simulink model "Client"  (R2021a)
settings: Solver=ode2  StartTime=0.0  StopTime=inf  FixedStep=0.002  RelTol=1e-3  EnableMultiTasking=on
libraries: quarc_library x19, simulink_extras x6, pid_lib x6, simulink x3
settings Model: SimulationMode=external  ExtModeTrigDuration=10000  Creator=user  LastModifiedBy=user
settings SolverCC: AlgebraicLoopSolver=TrustRegion  PositivePriorityOrder=on
settings DataIOCC: ReturnWorkspaceOutputs=off
settings DebuggingCC: SFMachineParentedDataDiag=warning  ArithmeticOperatorsInVariantConditions=warning
settings SFSimCC: SimUseLocalCustomCode=off  CustomCodeUndefinedFunction=UseInterfaceOnly
settings RTWCC: Description=QUARC Win64 Target Using Toolchain  SystemTargetFile=quarc_win64.tlc  TemplateMakefile=quarc_default_tmf  RTWUseLocalCustomCode=off  Toolchain=QUARC win64 | nmake (64-bit Windows)  BuildConfiguration=Faster Runs
settings CodeAppCC: StateflowObjectComments=on
settings STFCustomTargetCC: TargetLangStandard=C99 (ISO)  ConcurrentExecutionCompliant=on  SystemTargetFile=quarc_win64.tlc
settings GRTTargetCC: ParMdlRefBuildCompliant=off  CompOptLevelCompliant=off  CombineOutputUpdateFcns=off  MatFileLogging=off  CPPClassGenCompliant=off  GRTInterface=on  ExtMode=on  ExtModeMexFile=quarc_comm  ExtModeMexArgs='-w -d /tmp -uri %u','tcpip://localhost:17001'
settings ConfigComp: CovMetricSettings=dswe

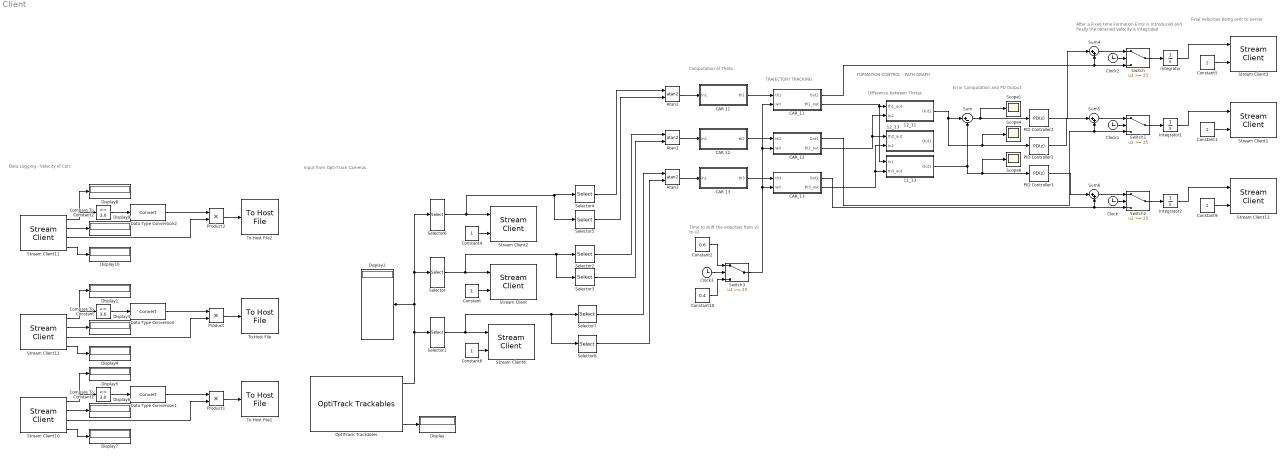
== system Client ==
  note: TRAJECTORY TRACKING
  note: FORMATION CONTROL - PATH GRAPH
  note: Difference between Thetas
  note: Error Computation and PD Output
  note: After a Fixed time Formation Error is
      | Introduced and finally the obtained
      | velocity is integrated
  note: Final Velocities being sent
      | to Server
  note: TIme to shift the velocities
      | from v1 to v2
  note: Computation of Theta
  note: Input from Opti-Track Cameras
  note: Data Logging - Velocity of Cars
  11_13 : Subsystem
  12_11 : Subsystem
  12_13 : Subsystem
  Atan1 : Trigonometry  Operator=atan2
  Atan2 : Trigonometry  Operator=atan2
  Atan3 : Trigonometry  Operator=atan2
  CAR 11 : Subsystem
  CAR 12 : Subsystem
  CAR 13 : Subsystem
  CAR_11 : Subsystem
  CAR_12 : Subsystem
  CAR_13 : Subsystem
  Clock{,1..3} (4 alike) : Clock
  Compare To Constant : simulink/Logic and Bit Operations/Compare To Constant  relop=<=  const=3.0  OutDataTypeStr=boolean
  Compare To Constant1 : simulink/Logic and Bit Operations/Compare To Constant  relop=<=  const=3.0  OutDataTypeStr=boolean
  Compare To Constant2 : simulink/Logic and Bit Operations/Compare To Constant  relop=<=  const=3.0  OutDataTypeStr=boolean
  Constant{,1,4..6,9} (6 alike) : Constant
  Constant10 : Constant  Value=0.4
  Constant2 : Constant  Value=0.6
  Data Type Conversion : DataTypeConversion
  Data Type Conversion1 : DataTypeConversion
  Data Type Conversion2 : DataTypeConversion
  Display{,1..10} (11 alike) : Display
  Integrator : Integrator  LimitOutput=on  UpperSaturationLimit=5  LowerSaturationLimit=0  WrappedStateUpperValue=5  WrappedStateLowerValue=0
  Integrator1 : Integrator  LimitOutput=on  UpperSaturationLimit=5  LowerSaturationLimit=0
  Integrator2 : Integrator  LimitOutput=on  UpperSaturationLimit=5  LowerSaturationLimit=0
  OptiTrack Trackables : quarc_library/Devices/Third-Party/NaturalPoint/OptiTrack/OptiTrack Trackables  calibration_file=C:\Users\user\Desktop\Motive_Calibration_SingleDrone\Camera_Calibration_Training\Calibration Exceptional (MeanErr 0.434 mm) 2023-02-26 3.cal  rigid_body_file=C:\Users\user\Desktop\Motive_Calibration_SingleDrone\Camera_Calibration_Training\3 Cars_1.tra  rigid_body_ids=[5 6 7]  sample_time=qc_get_step_size  active=off
      settings: SourceProductName=QUARC Targets
  PID Controller1 : pid_lib/PID Controller  Controller=PD  Form=Parallel  TimeDomain=Discrete-time  UseExternalTs=off  SampleTime=-1  IntegratorMethod=Forward Euler  FilterMethod=Forward Euler  ControllerParametersSource=internal  P=-0.68  I=-0.5  D=-1.75  UseFilter=on  N=1  TunerSelectOption=Transfer Function Based (PID Tuner App)  InitialConditionSource=internal  InitialConditionForIntegrator=0  InitialConditionForFilter=0  DifferentiatorICPrevScaledInput=0  ExternalReset=none  TrackingMode=off  Kt=1  LimitOutput=off  SatLimitsSource=internal  UpperSaturationLimit=inf  LowerSaturationLimit=-inf  LinearizeAsGain=on  AntiWindupMode=none  Kb=1  POutMin=[]  POutMax=[]  IOutMin=[]  IOutMax=[]  DOutMin=[]  DOutMax=[]  NOutMin=[]  NOutMax=[]  SumOutMin=[]  SumOutMax=[]  SaturationOutMin=[]  SaturationOutMax=[]  PParamMin=[]  PParamMax=[]  IParamMin=[]  IParamMax=[]  DParamMin=[]  DParamMax=[]  NParamMin=[]  NParamMax=[]  KbParamMin=[]  KbParamMax=[]  KtParamMin=[]  KtParamMax=[]  KbOutMin=[]  KbOutMax=[]  KtOutMin=[]  KtOutMax=[]  IntegratorOutMin=[]  IntegratorOutMax=[]  FilterOutMin=[]  FilterOutMax=[]  SumI1OutMin=[]  SumI1OutMax=[]  SumI2OutMin=[]  SumI2OutMax=[]  SumI3OutMin=[]  SumI3OutMax=[]  SumI4OutMin=[]  SumI4OutMax=[]  SumDOutMin=[]  SumDOutMax=[]  DifferentiatorOutMin=[]  DifferentiatorOutMax=[]  FilterDiffOutCoefMin=[]  FilterDiffOutCoefMax=[]  ReciprocalOutMin=[]  ReciprocalOutMax=[]  SumDenOutMin=[]  SumDenOutMax=[]  SumNumOutMin=[]  SumNumOutMax=[]  DivideOutMin=[]  DivideOutMax=[]  UdiffTsProdOutMin=[]  UdiffTsProdOutMax=[]  NTsProdOutMin=[]  NTsProdOutMax=[]  UintegralTsProdOutMin=[]  UintegralTsProdOutMax=[]  UngainTsProdOutMin=[]  UngainTsProdOutMax=[]  IntegratorContinuousStateAttributes=''  IntegratorStateMustResolveToSignalObject=off  IntegratorRTWStateStorageClass=Auto  FilterContinuousStateAttributes=''  FilterStateMustResolveToSignalObject=off  FilterRTWStateStorageClass=Auto  ParallelPVariant=InternalParameters  IdealPVariant=Disabled  IVariant=Disabled  DVariant=InternalParameters  IntegratorVariant=Disabled  SatVariant=Disabled  AWVariant=Disabled  PCopyVariant=Disabled  TRVariant=Disabled  FdbkBlocksVariant=Forward  IdealPFdbkVariant=Disabled  SatFdbkVariant=Disabled  DerivativeFilterVariant=ForwardEulerFilter  NVariant=InternalParameters  NCopyVariant=Disabled  FilterICVariant=InternalICsFilter  IntegratorICVariant=Disabled  ExternalResetVariant=Disabled  TRSumVariant=Passthrough  SumFdbkVariant=Disabled  SumVariant=Sum_PD  TsampFilterVariant=InternalTs  TsampNgainVariant=Passthrough  TsampIntegralVariant=Disabled_SignalSpec  ExternalSaturationOutDataTypeStr=Inherit: Same as second input
  PID Controller2 : pid_lib/PID Controller  Controller=PD  Form=Parallel  TimeDomain=Discrete-time  UseExternalTs=off  SampleTime=-1  IntegratorMethod=Forward Euler  FilterMethod=Forward Euler  ControllerParametersSource=internal  P=-0.68  I=-0.5  D=-1.75  UseFilter=on  N=1  TunerSelectOption=Transfer Function Based (PID Tuner App)  InitialConditionSource=internal  InitialConditionForIntegrator=0  InitialConditionForFilter=0  DifferentiatorICPrevScaledInput=0  ExternalReset=none  TrackingMode=off  Kt=1  LimitOutput=off  SatLimitsSource=internal  UpperSaturationLimit=inf  LowerSaturationLimit=-inf  LinearizeAsGain=on  AntiWindupMode=none  Kb=1  POutMin=[]  POutMax=[]  IOutMin=[]  IOutMax=[]  DOutMin=[]  DOutMax=[]  NOutMin=[]  NOutMax=[]  SumOutMin=[]  SumOutMax=[]  SaturationOutMin=[]  SaturationOutMax=[]  PParamMin=[]  PParamMax=[]  IParamMin=[]  IParamMax=[]  DParamMin=[]  DParamMax=[]  NParamMin=[]  NParamMax=[]  KbParamMin=[]  KbParamMax=[]  KtParamMin=[]  KtParamMax=[]  KbOutMin=[]  KbOutMax=[]  KtOutMin=[]  KtOutMax=[]  IntegratorOutMin=[]  IntegratorOutMax=[]  FilterOutMin=[]  FilterOutMax=[]  SumI1OutMin=[]  SumI1OutMax=[]  SumI2OutMin=[]  SumI2OutMax=[]  SumI3OutMin=[]  SumI3OutMax=[]  SumI4OutMin=[]  SumI4OutMax=[]  SumDOutMin=[]  SumDOutMax=[]  DifferentiatorOutMin=[]  DifferentiatorOutMax=[]  FilterDiffOutCoefMin=[]  FilterDiffOutCoefMax=[]  ReciprocalOutMin=[]  ReciprocalOutMax=[]  SumDenOutMin=[]  SumDenOutMax=[]  SumNumOutMin=[]  SumNumOutMax=[]  DivideOutMin=[]  DivideOutMax=[]  UdiffTsProdOutMin=[]  UdiffTsProdOutMax=[]  NTsProdOutMin=[]  NTsProdOutMax=[]  UintegralTsProdOutMin=[]  UintegralTsProdOutMax=[]  UngainTsProdOutMin=[]  UngainTsProdOutMax=[]  IntegratorContinuousStateAttributes=''  IntegratorStateMustResolveToSignalObject=off  IntegratorRTWStateStorageClass=Auto  FilterContinuousStateAttributes=''  FilterStateMustResolveToSignalObject=off  FilterRTWStateStorageClass=Auto  ParallelPVariant=InternalParameters  IdealPVariant=Disabled  IVariant=Disabled  DVariant=InternalParameters  IntegratorVariant=Disabled  SatVariant=Disabled  AWVariant=Disabled  PCopyVariant=Disabled  TRVariant=Disabled  FdbkBlocksVariant=Forward  IdealPFdbkVariant=Disabled  SatFdbkVariant=Disabled  DerivativeFilterVariant=ForwardEulerFilter  NVariant=InternalParameters  NCopyVariant=Disabled  FilterICVariant=InternalICsFilter  IntegratorICVariant=Disabled  ExternalResetVariant=Disabled  TRSumVariant=Passthrough  SumFdbkVariant=Disabled  SumVariant=Sum_PD  TsampFilterVariant=InternalTs  TsampNgainVariant=Passthrough  TsampIntegralVariant=Disabled_SignalSpec  ExternalSaturationOutDataTypeStr=Inherit: Same as second input
  PID Controller3 : pid_lib/PID Controller  Controller=PD  Form=Parallel  TimeDomain=Discrete-time  UseExternalTs=off  SampleTime=-1  IntegratorMethod=Forward Euler  FilterMethod=Forward Euler  ControllerParametersSource=internal  P=-0.68  I=-0.5  D=-1.75  UseFilter=on  N=1  TunerSelectOption=Transfer Function Based (PID Tuner App)  InitialConditionSource=internal  InitialConditionForIntegrator=0  InitialConditionForFilter=0  DifferentiatorICPrevScaledInput=0  ExternalReset=none  TrackingMode=off  Kt=1  LimitOutput=off  SatLimitsSource=internal  UpperSaturationLimit=inf  LowerSaturationLimit=-inf  LinearizeAsGain=on  AntiWindupMode=none  Kb=1  POutMin=[]  POutMax=[]  IOutMin=[]  IOutMax=[]  DOutMin=[]  DOutMax=[]  NOutMin=[]  NOutMax=[]  SumOutMin=[]  SumOutMax=[]  SaturationOutMin=[]  SaturationOutMax=[]  PParamMin=[]  PParamMax=[]  IParamMin=[]  IParamMax=[]  DParamMin=[]  DParamMax=[]  NParamMin=[]  NParamMax=[]  KbParamMin=[]  KbParamMax=[]  KtParamMin=[]  KtParamMax=[]  KbOutMin=[]  KbOutMax=[]  KtOutMin=[]  KtOutMax=[]  IntegratorOutMin=[]  IntegratorOutMax=[]  FilterOutMin=[]  FilterOutMax=[]  SumI1OutMin=[]  SumI1OutMax=[]  SumI2OutMin=[]  SumI2OutMax=[]  SumI3OutMin=[]  SumI3OutMax=[]  SumI4OutMin=[]  SumI4OutMax=[]  SumDOutMin=[]  SumDOutMax=[]  DifferentiatorOutMin=[]  DifferentiatorOutMax=[]  FilterDiffOutCoefMin=[]  FilterDiffOutCoefMax=[]  ReciprocalOutMin=[]  ReciprocalOutMax=[]  SumDenOutMin=[]  SumDenOutMax=[]  SumNumOutMin=[]  SumNumOutMax=[]  DivideOutMin=[]  DivideOutMax=[]  UdiffTsProdOutMin=[]  UdiffTsProdOutMax=[]  NTsProdOutMin=[]  NTsProdOutMax=[]  UintegralTsProdOutMin=[]  UintegralTsProdOutMax=[]  UngainTsProdOutMin=[]  UngainTsProdOutMax=[]  IntegratorContinuousStateAttributes=''  IntegratorStateMustResolveToSignalObject=off  IntegratorRTWStateStorageClass=Auto  FilterContinuousStateAttributes=''  FilterStateMustResolveToSignalObject=off  FilterRTWStateStorageClass=Auto  ParallelPVariant=InternalParameters  IdealPVariant=Disabled  IVariant=Disabled  DVariant=InternalParameters  IntegratorVariant=Disabled  SatVariant=Disabled  AWVariant=Disabled  PCopyVariant=Disabled  TRVariant=Disabled  FdbkBlocksVariant=Forward  IdealPFdbkVariant=Disabled  SatFdbkVariant=Disabled  DerivativeFilterVariant=ForwardEulerFilter  NVariant=InternalParameters  NCopyVariant=Disabled  FilterICVariant=InternalICsFilter  IntegratorICVariant=Disabled  ExternalResetVariant=Disabled  TRSumVariant=Passthrough  SumFdbkVariant=Disabled  SumVariant=Sum_PD  TsampFilterVariant=InternalTs  TsampNgainVariant=Passthrough  TsampIntegralVariant=Disabled_SignalSpec  ExternalSaturationOutDataTypeStr=Inherit: Same as second input
  Product : Product
  Product1 : Product
  Product2 : Product
  Scope1 : Scope
  Scope4 : Scope
  Scope6 : Scope
  Selector : Selector  InputPortWidth=9  IndexOptions=Index vector (dialog)  Indices=[1 3]  OutputSizes=1
  Selector1 : Selector  InputPortWidth=9  IndexOptions=Index vector (dialog)  Indices=[7 9]  OutputSizes=1
  Selector2 : Selector  InputPortWidth=2  IndexOptions=Index vector (dialog)  Indices=[1]  OutputSizes=1
  Selector3 : Selector  InputPortWidth=2  IndexOptions=Index vector (dialog)  Indices=[2]  OutputSizes=1
  Selector4 : Selector  InputPortWidth=2  IndexOptions=Index vector (dialog)  Indices=[1]  OutputSizes=1
  Selector5 : Selector  InputPortWidth=2  IndexOptions=Index vector (dialog)  Indices=[2]  OutputSizes=1
  Selector6 : Selector  InputPortWidth=9  IndexOptions=Index vector (dialog)  Indices=[4 6]  OutputSizes=1
  Selector7 : Selector  InputPortWidth=2  IndexOptions=Index vector (dialog)  Indices=[1]  OutputSizes=1
  Selector8 : Selector  InputPortWidth=2  IndexOptions=Index vector (dialog)  Indices=[2]  OutputSizes=1
  Stream Client : quarc_library/Communications/Basic/Stream Client  uri_source=Specify via dialog (do not evaluate)  uri=tcpip://192.168.2.12:18070  send_buffer_size=1460  receive_buffer_size=1460  byte_order=little endian (Intel - LSB first)  optimization=Minimum latency  send_options=Send most recent data  receive_options=Do not receive data  default_value=[0]  sample_time=qc_get_step_size  active=off  implementation=Use blocking I/O in a separate thread  send_fifo_size=1000  receive_fifo_size=1000  send_priority=0  receive_priority=0  send_dimensions=off  receive_dimensions=off  max_dimensions=-1  data_type=Inherited via back propagation  type_expr=BusObject
      settings: AttributesFormatString="\"tcpip://192.168.2.12:18070\""
  Stream Client1 : quarc_library/Communications/Basic/Stream Client  uri_source=Specify via dialog (do not evaluate)  uri=tcpip://192.168.2.12:18071  send_buffer_size=1460  receive_buffer_size=1460  byte_order=little endian (Intel - LSB first)  optimization=Minimum latency  send_options=Send most recent data  receive_options=Do not receive data  default_value=[0]  sample_time=qc_get_step_size  active=off  implementation=Use blocking I/O in a separate thread  send_fifo_size=1000  receive_fifo_size=1000  send_priority=0  receive_priority=0  send_dimensions=off  receive_dimensions=off  max_dimensions=-1  data_type=Inherited via back propagation  type_expr=BusObject
      settings: AttributesFormatString="\"tcpip://192.168.2.12:18071\""
  Stream Client10 : quarc_library/Communications/Basic/Stream Client  uri_source=Specify via dialog (do not evaluate)  uri=tcpip://192.168.2.12:18099  send_buffer_size=1460  receive_buffer_size=1460  byte_order=little endian (Intel - LSB first)  optimization=Minimum latency  send_options=Do not send data  receive_options=Receive most recent data  default_value=[0]  sample_time=qc_get_step_size  active=off  implementation=Use blocking I/O in a separate thread  send_fifo_size=1000  receive_fifo_size=1000  send_priority=0  receive_priority=0  send_dimensions=off  receive_dimensions=off  max_dimensions=-1  data_type=Inherited via back propagation  type_expr=BusObject
      settings: AttributesFormatString="\"tcpip://192.168.2.12:18099\""
  Stream Client11 : quarc_library/Communications/Basic/Stream Client  uri_source=Specify via dialog (do not evaluate)  uri=tcpip://192.168.2.13:18079  send_buffer_size=1460  receive_buffer_size=1460  byte_order=little endian (Intel - LSB first)  optimization=Minimum latency  send_options=Do not send data  receive_options=Receive most recent data  default_value=[0]  sample_time=qc_get_step_size  active=off  implementation=Use blocking I/O in a separate thread  send_fifo_size=1000  receive_fifo_size=1000  send_priority=0  receive_priority=0  send_dimensions=off  receive_dimensions=off  max_dimensions=-1  data_type=Inherited via back propagation  type_expr=BusObject
      settings: AttributesFormatString="\"tcpip://192.168.2.13:18079\""
  Stream Client12 : quarc_library/Communications/Basic/Stream Client  uri_source=Specify via dialog (do not evaluate)  uri=tcpip://192.168.2.11:18089  send_buffer_size=1460  receive_buffer_size=1460  byte_order=little endian (Intel - LSB first)  optimization=Minimum latency  send_options=Do not send data  receive_options=Receive most recent data  default_value=[0]  sample_time=qc_get_step_size  active=off  implementation=Use blocking I/O in a separate thread  send_fifo_size=1000  receive_fifo_size=1000  send_priority=0  receive_priority=0  send_dimensions=off  receive_dimensions=off  max_dimensions=-1  data_type=Inherited via back propagation  type_expr=BusObject
      settings: AttributesFormatString="\"tcpip://192.168.2.11:18089\""
  Stream Client13 : quarc_library/Communications/Basic/Stream Client  uri_source=Specify via dialog (do not evaluate)  uri=tcpip://192.168.2.13:18091  send_buffer_size=1460  receive_buffer_size=1460  byte_order=little endian (Intel - LSB first)  optimization=Minimum latency  send_options=Send most recent data  receive_options=Do not receive data  default_value=[0]  sample_time=qc_get_step_size  active=off  implementation=Use blocking I/O in a separate thread  send_fifo_size=1000  receive_fifo_size=1000  send_priority=0  receive_priority=0  send_dimensions=off  receive_dimensions=off  max_dimensions=-1  data_type=Inherited via back propagation  type_expr=BusObject
      settings: AttributesFormatString="\"tcpip://192.168.2.13:18091\""
  Stream Client2 : quarc_library/Communications/Basic/Stream Client  uri_source=Specify via dialog (do not evaluate)  uri=tcpip://192.168.2.11:18080  send_buffer_size=1460  receive_buffer_size=1460  byte_order=little endian (Intel - LSB first)  optimization=Minimum latency  send_options=Send most recent data  receive_options=Do not receive data  default_value=[0]  sample_time=qc_get_step_size  active=off  implementation=Use blocking I/O in a separate thread  send_fifo_size=1000  receive_fifo_size=1000  send_priority=0  receive_priority=0  send_dimensions=off  receive_dimensions=off  max_dimensions=-1  data_type=Inherited via back propagation  type_expr=BusObject
      settings: AttributesFormatString="\"tcpip://192.168.2.11:18080\""
  Stream Client3 : quarc_library/Communications/Basic/Stream Client  uri_source=Specify via dialog (do not evaluate)  uri=tcpip://192.168.2.11:18081  send_buffer_size=1460  receive_buffer_size=1460  byte_order=little endian (Intel - LSB first)  optimization=Minimum latency  send_options=Send most recent data  receive_options=Do not receive data  default_value=[0]  sample_time=qc_get_step_size  active=off  implementation=Use blocking I/O in a separate thread  send_fifo_size=1000  receive_fifo_size=1000  send_priority=0  receive_priority=0  send_dimensions=off  receive_dimensions=off  max_dimensions=-1  data_type=Inherited via back propagation  type_expr=BusObject
      settings: AttributesFormatString="\"tcpip://192.168.2.11:18081\""
  Stream Client6 : quarc_library/Communications/Basic/Stream Client  uri_source=Specify via dialog (do not evaluate)  uri=tcpip://192.168.2.13:18090  send_buffer_size=1460  receive_buffer_size=1460  byte_order=little endian (Intel - LSB first)  optimization=Minimum latency  send_options=Send most recent data  receive_options=Do not receive data  default_value=[0]  sample_time=qc_get_step_size  active=off  implementation=Use blocking I/O in a separate thread  send_fifo_size=1000  receive_fifo_size=1000  send_priority=0  receive_priority=0  send_dimensions=off  receive_dimensions=off  max_dimensions=-1  data_type=Inherited via back propagation  type_expr=BusObject
      settings: AttributesFormatString="\"tcpip://192.168.2.13:18090\""
  Sum : Sum  Inputs=|+-
  Sum4 : Sum  Inputs=|++
  Sum5 : Sum  Inputs=|++
  Sum6 : Sum  Inputs=|++
  Switch{,1..3} (4 alike) : Switch  Threshold=25
  To Host File : quarc_library/Sinks/To Host/To Host File  file_name=data_v_11.mat  variable_name=data_v_11  decimation=1  sample_time=-1  file_format=MAT-file v.4  options=No header or footer  append=off  final_file_name=data_v_11.mat  bitrate=2000000
  To Host File1 : quarc_library/Sinks/To Host/To Host File  file_name=data_v_12.mat  variable_name=data_v_12  decimation=1  sample_time=-1  file_format=MAT-file v.4  options=No header or footer  append=off  final_file_name=data_v_12.mat  bitrate=2000000
  To Host File2 : quarc_library/Sinks/To Host/To Host File  file_name=data_v_13.mat  variable_name=data_v_13  decimation=1  sample_time=-1  file_format=MAT-file v.4  options=No header or footer  append=off  final_file_name=data_v_13.mat  bitrate=2000000
  wires:
  OptiTrack Trackables/4 -> Display/1
  OptiTrack Trackables/1 -> Display2/1, Selector6/1, Selector/1, Selector1/1
  Constant/1 -> Stream Client/2
  Constant1/1 -> Stream Client1/2
  Constant5/1 -> Stream Client3/2
  Constant4/1 -> Stream Client2/2
  Selector1/1 -> Stream Client6/1, Selector7/1, Selector8/1
  Constant6/1 -> Stream Client6/2
  Constant9/1 -> Stream Client13/2
  Stream Client12/1 -> Display1/1, Compare To Constant/1
  Stream Client11/4 -> Display10/1
  Data Type Conversion2/1 -> Product2/1
  Product2/1 -> To Host File2/1
  Compare To Constant1/1 -> Data Type Conversion1/1
  Stream Client11/2 -> Display9/1
  Product/1 -> To Host File/1
  Data Type Conversion1/1 -> Product1/1
  Stream Client11/3 -> Product2/2
  Compare To Constant2/1 -> Data Type Conversion2/1
  Stream Client12/4 -> Display4/1
  Stream Client10/2 -> Display6/1
  Stream Client11/1 -> Display8/1, Compare To Constant2/1
  Stream Client10/3 -> Product1/2
  Stream Client12/3 -> Product/2
  Stream Client12/2 -> Display3/1
  Product1/1 -> To Host File1/1
  Data Type Conversion/1 -> Product/1
  Stream Client10/4 -> Display7/1
  Compare To Constant/1 -> Data Type Conversion/1
  Stream Client10/1 -> Compare To Constant1/1, Display5/1
  Selector8/1 -> Atan3/2
  Selector7/1 -> Atan3/1
  Selector3/1 -> Atan1/2
  Selector/1 -> Stream Client/1, Selector3/1, Selector2/1
  Selector2/1 -> Atan1/1
  Selector5/1 -> Atan2/2
  Selector4/1 -> Atan2/1
  Selector6/1 -> Selector5/1, Selector4/1, Stream Client2/1
  Atan2/1 -> CAR 11/1(In1)
  Atan3/1 -> CAR 13/1(In1)
  Atan1/1 -> CAR 12/1(In1)
  Switch3/1 -> CAR_13/2(wd), CAR_12/2(wd), CAR_11/2(wd)
  CAR 12/1(th2) -> CAR_12/1(th2)
  CAR 11/1(th1) -> CAR_11/1(th1)
  CAR 13/1(th3) -> CAR_13/1(th3)
  CAR_11/2(th1_out) -> 11_13/1(In1), 12_11/1(th1_out)
  CAR_12/2(th2_out) -> 12_13/1(th2_out), 12_11/2(In2)
  CAR_13/2(th3_out) -> 11_13/2(th3_out), 12_13/2(In2)
  Sum/1 -> Scope1/1, PID Controller2/1
  Clock/1 -> Switch2/2
  Clock1/1 -> Switch1/2
  Clock2/1 -> Switch/2
  CAR_11/1(Out1) -> Sum4/2, Switch/3
  CAR_13/1(Out1) -> Sum6/2, Switch2/3
  Sum4/1 -> Switch/1
  Sum5/1 -> Switch1/1
  Sum6/1 -> Switch2/1
  Constant10/1 -> Switch3/3
  Constant2/1 -> Switch3/1
  Clock3/1 -> Switch3/2
  CAR_12/1(Out1) -> Switch1/3, Sum5/2
  Switch/1 -> Integrator/1
  Switch1/1 -> Integrator1/1
  Switch2/1 -> Integrator2/1
  Integrator/1 -> Stream Client3/1
  Integrator1/1 -> Stream Client1/1
  Integrator2/1 -> Stream Client13/1
  12_11/1(Out1) -> Sum/1, PID Controller1/1, Scope4/1
  11_13/1(Out1) -> PID Controller3/1, Scope6/1, Sum/2
  PID Controller2/1 -> Sum4/1
  PID Controller1/1 -> Sum5/1
  PID Controller3/1 -> Sum6/1

== system Client/11_13 ==
  In1 : Inport
  th3_out : Inport  Port=2
  Constant : Constant  Value=2.0943951
  Scope : Scope
  Sum : Sum  Inputs=|-+
  Sum1 : Sum  Inputs=|+-
  Out1 : Outport
  wires:
  th3_out/1 -> Sum/2
  In1/1 -> Sum/1
  Sum1/1 -> Scope/1, Out1/1
  Constant/1 -> Sum1/2
  Sum/1 -> Sum1/1

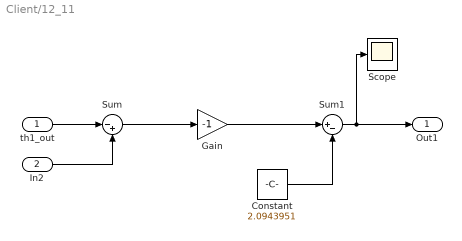
== system Client/12_11 ==
  th1_out : Inport
  In2 : Inport  Port=2
  Constant : Constant  Value=2.0943951
  Gain : Gain  Gain=-1
  Scope : Scope
  Sum : Sum  Inputs=|-+
  Sum1 : Sum  Inputs=|+-
  Out1 : Outport
  wires:
  th1_out/1 -> Sum/1
  In2/1 -> Sum/2
  Sum/1 -> Gain/1
  Gain/1 -> Sum1/1
  Sum1/1 -> Scope/1, Out1/1
  Constant/1 -> Sum1/2

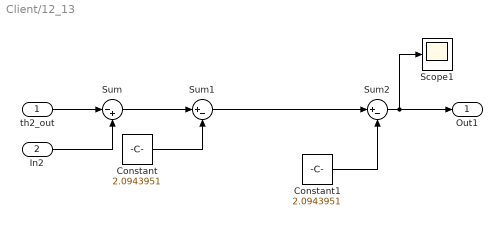
== system Client/12_13 ==
  th2_out : Inport
  In2 : Inport  Port=2
  Constant : Constant  Value=2.0943951
  Constant1 : Constant  Value=2.0943951
  Scope1 : Scope
  Sum : Sum  Inputs=|-+
  Sum1 : Sum  Inputs=|+-
  Sum2 : Sum  Inputs=|+-
  Out1 : Outport
  wires:
  Sum/1 -> Sum1/1
  In2/1 -> Sum/2
  th2_out/1 -> Sum/1
  Constant/1 -> Sum1/2
  Sum2/1 -> Scope1/1, Out1/1
  Constant1/1 -> Sum2/2
  Sum1/1 -> Sum2/1

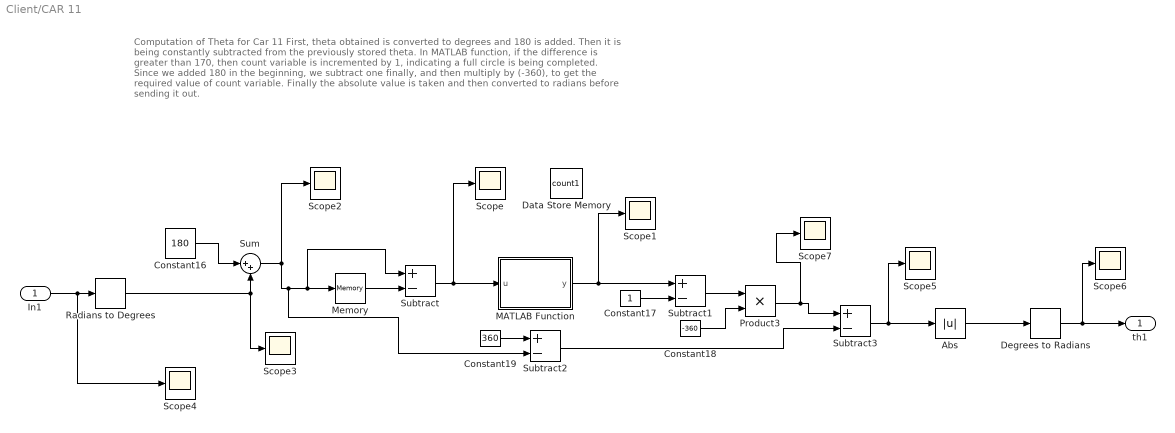
== system Client/CAR 11 ==
  note: Computation of Theta for Car 11
      | First, theta obtained is converted to degrees and 180 is added.
      | Then it is being constantly subtracted from the previously stored theta.
      | In MATLAB function, if the difference is greater than 170, then count variable is incremented by 1, indicating a full circle is being completed.
      | Since we added 180 in the beginning, we subtract one finally, and then multiply by (-360), to get the required value of count variable.
      | Finally the absolute value is taken and then converted to radians before sending it out.
  In1 : Inport
  Abs : Abs
  Constant16 : Constant  Value=180
  Constant17 : Constant
  Constant18 : Constant  Value=-360
  Constant19 : Constant  Value=360
  Data Store Memory : DataStoreMemory  DataStoreName=count1  ReadBeforeWriteMsg=warning  WriteAfterWriteMsg=warning  WriteAfterReadMsg=warning  ShowAdditionalParam=off  OutMin=0  OutDataTypeStr=double
  Degrees to Radians : simulink_extras/Transformations/Degrees to Radians
  MATLAB Function : MATLAB Function  TreatAsAtomicUnit=on
  Memory : Memory
  Product3 : Product
  Radians to Degrees : simulink_extras/Transformations/Radians to Degrees
  Scope{,1..7} (8 alike) : Scope
  Subtract{,1..3} (4 alike) : Sum  Inputs=+-
  Sum : Sum  Inputs=|++
  th1 : Outport
  wires:
  Constant16/1 -> Sum/1
  MATLAB Function/1(y) -> Scope1/1, Subtract1/1
  Subtract/1 -> Scope/1, MATLAB Function/1(u)
  Memory/1 -> Subtract/2
  Sum/1 -> Subtract2/2, Subtract/1, Memory/1, Scope2/1
  Constant17/1 -> Subtract1/2
  Subtract3/1 -> Abs/1, Scope5/1
  Product3/1 -> Scope7/1, Subtract3/1
  Subtract2/1 -> Subtract3/2
  Constant18/1 -> Product3/2
  Constant19/1 -> Subtract2/1
  In1/1 -> Radians to Degrees/1, Scope4/1
  Subtract1/1 -> Product3/1
  Abs/1 -> Degrees to Radians/1
  Degrees to Radians/1 -> Scope6/1, th1/1
  Radians to Degrees/1 -> Sum/2, Scope3/1

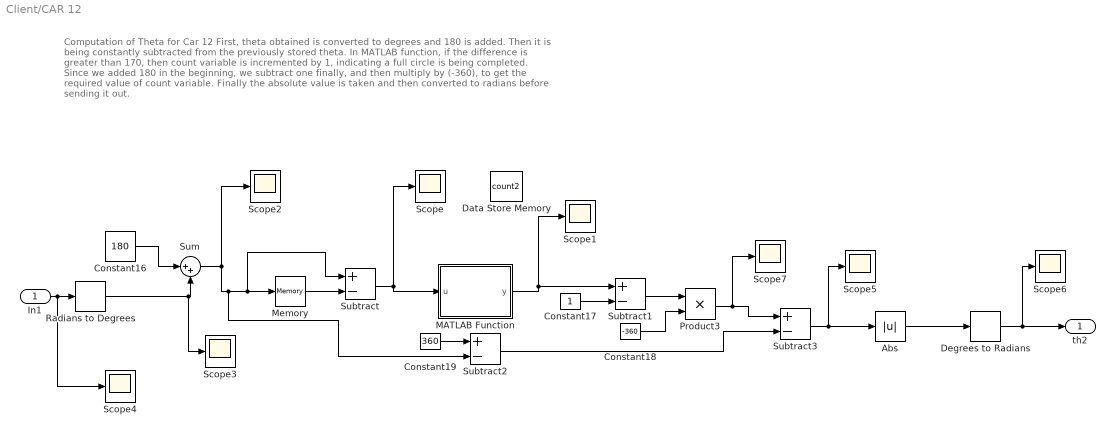
== system Client/CAR 12 ==
  note: Computation of Theta for Car 12
      | First, theta obtained is converted to degrees and 180 is added.
      | Then it is being constantly subtracted from the previously stored theta.
      | In MATLAB function, if the difference is greater than 170, then count variable is incremented by 1, indicating a full circle is being completed.
      | Since we added 180 in the beginning, we subtract one finally, and then multiply by (-360), to get the required value of count variable.
      | Finally the absolute value is taken and then converted to radians before sending it out.
  In1 : Inport
  Abs : Abs
  Constant16 : Constant  Value=180
  Constant17 : Constant
  Constant18 : Constant  Value=-360
  Constant19 : Constant  Value=360
  Data Store Memory : DataStoreMemory  DataStoreName=count2  ReadBeforeWriteMsg=warning  WriteAfterWriteMsg=warning  WriteAfterReadMsg=warning  ShowAdditionalParam=off  OutMin=0  OutDataTypeStr=double
  Degrees to Radians : simulink_extras/Transformations/Degrees to Radians
  MATLAB Function : MATLAB Function  TreatAsAtomicUnit=on
  Memory : Memory
  Product3 : Product
  Radians to Degrees : simulink_extras/Transformations/Radians to Degrees
  Scope{,1..7} (8 alike) : Scope
  Subtract{,1..3} (4 alike) : Sum  Inputs=+-
  Sum : Sum  Inputs=|++
  th2 : Outport
  wires:
  Degrees to Radians/1 -> th2/1, Scope6/1
  Abs/1 -> Degrees to Radians/1
  Subtract1/1 -> Product3/1
  In1/1 -> Radians to Degrees/1, Scope4/1
  Constant19/1 -> Subtract2/1
  Constant18/1 -> Product3/2
  Subtract2/1 -> Subtract3/2
  Product3/1 -> Scope7/1, Subtract3/1
  Subtract3/1 -> Scope5/1, Abs/1
  Constant17/1 -> Subtract1/2
  Sum/1 -> Scope2/1, Memory/1, Subtract/1, Subtract2/2
  Memory/1 -> Subtract/2
  Subtract/1 -> MATLAB Function/1(u), Scope/1
  MATLAB Function/1(y) -> Subtract1/1, Scope1/1
  Constant16/1 -> Sum/1
  Radians to Degrees/1 -> Scope3/1, Sum/2

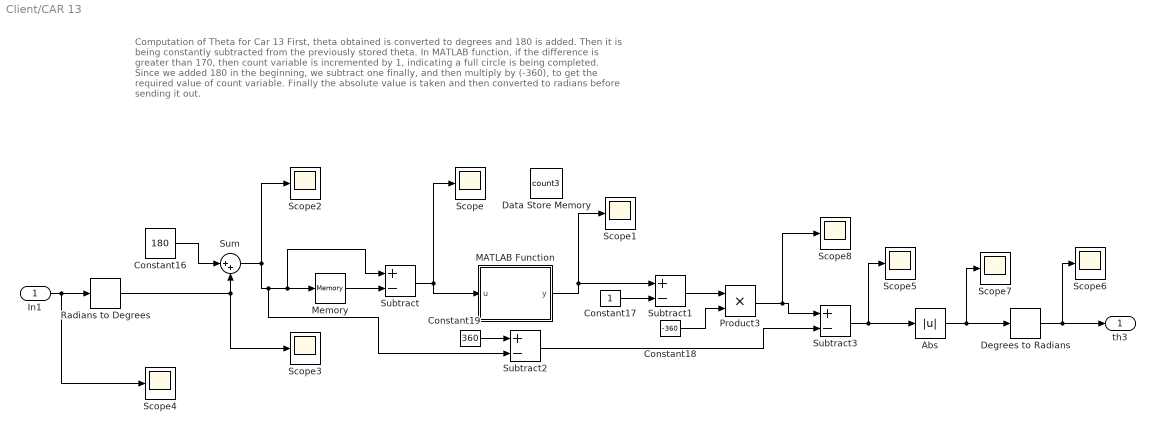
== system Client/CAR 13 ==
  note: Computation of Theta for Car 13
      | First, theta obtained is converted to degrees and 180 is added.
      | Then it is being constantly subtracted from the previously stored theta.
      | In MATLAB function, if the difference is greater than 170, then count variable is incremented by 1, indicating a full circle is being completed.
      | Since we added 180 in the beginning, we subtract one finally, and then multiply by (-360), to get the required value of count variable.
      | Finally the absolute value is taken and then converted to radians before sending it out.
  In1 : Inport
  Abs : Abs
  Constant16 : Constant  Value=180
  Constant17 : Constant
  Constant18 : Constant  Value=-360
  Constant19 : Constant  Value=360
  Data Store Memory : DataStoreMemory  DataStoreName=count3  ReadBeforeWriteMsg=warning  WriteAfterWriteMsg=warning  WriteAfterReadMsg=warning  ShowAdditionalParam=off  OutMin=0  OutDataTypeStr=double
  Degrees to Radians : simulink_extras/Transformations/Degrees to Radians
  MATLAB Function : MATLAB Function  TreatAsAtomicUnit=on
  Memory : Memory
  Product3 : Product
  Radians to Degrees : simulink_extras/Transformations/Radians to Degrees
  Scope{,1..8} (9 alike) : Scope
  Subtract{,1..3} (4 alike) : Sum  Inputs=+-
  Sum : Sum  Inputs=|++
  th3 : Outport
  wires:
  Constant16/1 -> Sum/1
  MATLAB Function/1(y) -> Scope1/1, Subtract1/1
  Subtract/1 -> Scope/1, MATLAB Function/1(u)
  Memory/1 -> Subtract/2
  Sum/1 -> Subtract2/2, Subtract/1, Memory/1, Scope2/1
  Constant17/1 -> Subtract1/2
  Subtract3/1 -> Abs/1, Scope5/1
  Product3/1 -> Scope8/1, Subtract3/1
  Subtract2/1 -> Subtract3/2
  Constant18/1 -> Product3/2
  Constant19/1 -> Subtract2/1
  In1/1 -> Radians to Degrees/1, Scope4/1
  Subtract1/1 -> Product3/1
  Abs/1 -> Scope7/1, Degrees to Radians/1
  Degrees to Radians/1 -> Scope6/1, th3/1
  Radians to Degrees/1 -> Scope3/1, Sum/2

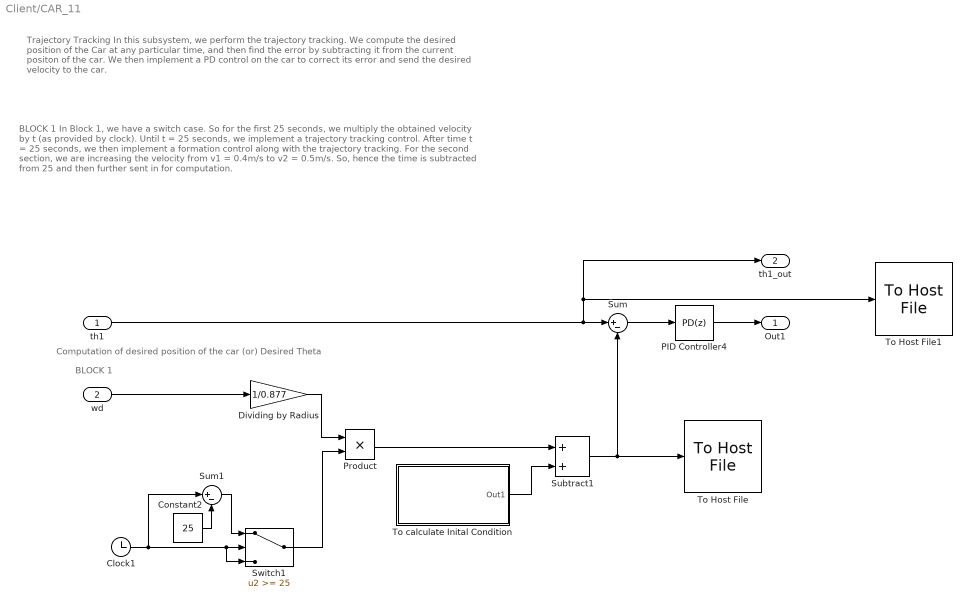
== system Client/CAR_11 ==
  note: Trajectory Tracking
      | In this subsystem, we perform the trajectory tracking.
      | We compute the desired position of the Car at any particular time, and then find the error by subtracting it from the current positon of the car.
      | We then implement a PD control on the car to correct its error and send the desired velocity to the car.
  note: BLOCK 1
  note: BLOCK 1
      | In Block 1, we have a switch case.
      | So for the first 25 seconds, we multiply the obtained velocity by t (as provided by clock). Until t = 25 seconds, we implement a trajectory tracking control.
      | After time t = 25 seconds, we then implement a formation control along with the trajectory tracking.
      | For the second section, we are increasing the velocity from v1 = 0.4m/s to v2 = 0.5m/s.
      | So, hence the time is subtracted from 25 and then further sent in for computation.
  note: Computation of desired position of the car (or) Desired Theta
  th1 : Inport
  wd : Inport  Port=2
  Clock1 : Clock
  Constant2 : Constant  Value=25
  Dividing by Radius : Gain  Gain=1/0.877
  PID Controller4 : pid_lib/PID Controller  Controller=PD  Form=Parallel  TimeDomain=Discrete-time  UseExternalTs=off  SampleTime=-1  IntegratorMethod=Forward Euler  FilterMethod=Forward Euler  ControllerParametersSource=internal  P=-0.68  I=-0.5  D=-1.75  UseFilter=on  N=1  TunerSelectOption=Transfer Function Based (PID Tuner App)  InitialConditionSource=internal  InitialConditionForIntegrator=0  InitialConditionForFilter=0  DifferentiatorICPrevScaledInput=0  ExternalReset=none  TrackingMode=off  Kt=1  LimitOutput=off  SatLimitsSource=internal  UpperSaturationLimit=inf  LowerSaturationLimit=-inf  LinearizeAsGain=on  AntiWindupMode=none  Kb=1  POutMin=[]  POutMax=[]  IOutMin=[]  IOutMax=[]  DOutMin=[]  DOutMax=[]  NOutMin=[]  NOutMax=[]  SumOutMin=[]  SumOutMax=[]  SaturationOutMin=[]  SaturationOutMax=[]  PParamMin=[]  PParamMax=[]  IParamMin=[]  IParamMax=[]  DParamMin=[]  DParamMax=[]  NParamMin=[]  NParamMax=[]  KbParamMin=[]  KbParamMax=[]  KtParamMin=[]  KtParamMax=[]  KbOutMin=[]  KbOutMax=[]  KtOutMin=[]  KtOutMax=[]  IntegratorOutMin=[]  IntegratorOutMax=[]  FilterOutMin=[]  FilterOutMax=[]  SumI1OutMin=[]  SumI1OutMax=[]  SumI2OutMin=[]  SumI2OutMax=[]  SumI3OutMin=[]  SumI3OutMax=[]  SumI4OutMin=[]  SumI4OutMax=[]  SumDOutMin=[]  SumDOutMax=[]  DifferentiatorOutMin=[]  DifferentiatorOutMax=[]  FilterDiffOutCoefMin=[]  FilterDiffOutCoefMax=[]  ReciprocalOutMin=[]  ReciprocalOutMax=[]  SumDenOutMin=[]  SumDenOutMax=[]  SumNumOutMin=[]  SumNumOutMax=[]  DivideOutMin=[]  DivideOutMax=[]  UdiffTsProdOutMin=[]  UdiffTsProdOutMax=[]  NTsProdOutMin=[]  NTsProdOutMax=[]  UintegralTsProdOutMin=[]  UintegralTsProdOutMax=[]  UngainTsProdOutMin=[]  UngainTsProdOutMax=[]  IntegratorContinuousStateAttributes=''  IntegratorStateMustResolveToSignalObject=off  IntegratorRTWStateStorageClass=Auto  FilterContinuousStateAttributes=''  FilterStateMustResolveToSignalObject=off  FilterRTWStateStorageClass=Auto  ParallelPVariant=InternalParameters  IdealPVariant=Disabled  IVariant=Disabled  DVariant=InternalParameters  IntegratorVariant=Disabled  SatVariant=Disabled  AWVariant=Disabled  PCopyVariant=Disabled  TRVariant=Disabled  FdbkBlocksVariant=Forward  IdealPFdbkVariant=Disabled  SatFdbkVariant=Disabled  DerivativeFilterVariant=ForwardEulerFilter  NVariant=InternalParameters  NCopyVariant=Disabled  FilterICVariant=InternalICsFilter  IntegratorICVariant=Disabled  ExternalResetVariant=Disabled  TRSumVariant=Passthrough  SumFdbkVariant=Disabled  SumVariant=Sum_PD  TsampFilterVariant=InternalTs  TsampNgainVariant=Passthrough  TsampIntegralVariant=Disabled_SignalSpec  ExternalSaturationOutDataTypeStr=Inherit: Same as second input
  Product : Product
  Subtract1 : Sum
  Sum : Sum  Inputs=|+-
  Sum1 : Sum  Inputs=|+-
  Switch1 : Switch  Threshold=25
  To Host File : quarc_library/Sinks/To Host/To Host File  file_name=CAR_11_Desired.mat  variable_name=CAR_11_Desired  decimation=1  sample_time=-1  file_format=MAT-file v.4  options=No header or footer  append=off  final_file_name=CAR_11_Desired.mat  bitrate=2000000
  To Host File1 : quarc_library/Sinks/To Host/To Host File  file_name=CAR_11_obtained.mat  variable_name=CAR_11_obtained  decimation=1  sample_time=-1  file_format=MAT-file v.4  options=No header or footer  append=off  final_file_name=CAR_11_obtained.mat  bitrate=2000000
  To calculate Inital Condition : Subsystem
  Out1 : Outport
  th1_out : Outport  Port=2
  wires:
  Subtract1/1 -> Sum/2, To Host File/1
  To calculate Inital Condition/1(Out1) -> Subtract1/2
  th1/1 -> Sum/1, th1_out/1, To Host File1/1
  Product/1 -> Subtract1/1
  Switch1/1 -> Product/2
  Dividing by Radius/1 -> Product/1
  Sum1/1 -> Switch1/1
  wd/1 -> Dividing by Radius/1
  Clock1/1 -> Switch1/3, Switch1/2, Sum1/1
  PID Controller4/1 -> Out1/1
  Sum/1 -> PID Controller4/1
  Constant2/1 -> Sum1/2

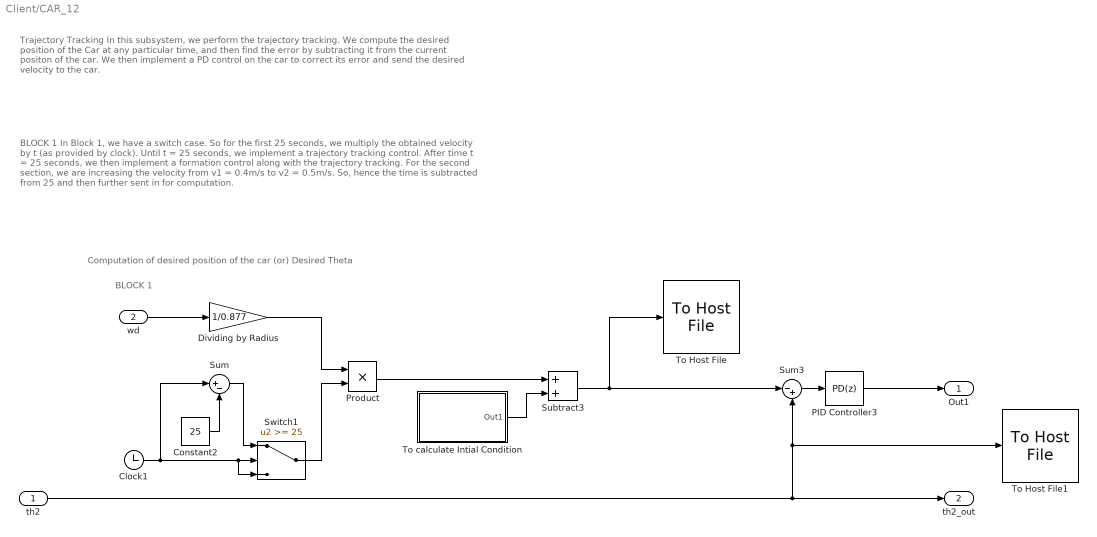
== system Client/CAR_12 ==
  note: BLOCK 1
      | In Block 1, we have a switch case.
      | So for the first 25 seconds, we multiply the obtained velocity by t (as provided by clock). Until t = 25 seconds, we implement a trajectory tracking control.
      | After time t = 25 seconds, we then implement a formation control along with the trajectory tracking.
      | For the second section, we are increasing the velocity from v1 = 0.4m/s to v2 = 0.5m/s.
      | So, hence the time is subtracted from 25 and then further sent in for computation.
  note: Trajectory Tracking
      | In this subsystem, we perform the trajectory tracking.
      | We compute the desired position of the Car at any particular time, and then find the error by subtracting it from the current positon of the car.
      | We then implement a PD control on the car to correct its error and send the desired velocity to the car.
  note: Computation of desired position of the car (or) Desired Theta
  note: BLOCK 1
  th2 : Inport
  wd : Inport  Port=2
  Clock1 : Clock
  Constant2 : Constant  Value=25
  Dividing by Radius : Gain  Gain=1/0.877
  PID Controller3 : pid_lib/PID Controller  Controller=PD  Form=Parallel  TimeDomain=Discrete-time  UseExternalTs=off  SampleTime=-1  IntegratorMethod=Forward Euler  FilterMethod=Forward Euler  ControllerParametersSource=internal  P=-0.68  I=-0.5  D=-1.75  UseFilter=on  N=1  TunerSelectOption=Transfer Function Based (PID Tuner App)  InitialConditionSource=internal  InitialConditionForIntegrator=0  InitialConditionForFilter=0  DifferentiatorICPrevScaledInput=0  ExternalReset=none  TrackingMode=off  Kt=1  LimitOutput=off  SatLimitsSource=internal  UpperSaturationLimit=inf  LowerSaturationLimit=-inf  LinearizeAsGain=on  AntiWindupMode=none  Kb=1  POutMin=[]  POutMax=[]  IOutMin=[]  IOutMax=[]  DOutMin=[]  DOutMax=[]  NOutMin=[]  NOutMax=[]  SumOutMin=[]  SumOutMax=[]  SaturationOutMin=[]  SaturationOutMax=[]  PParamMin=[]  PParamMax=[]  IParamMin=[]  IParamMax=[]  DParamMin=[]  DParamMax=[]  NParamMin=[]  NParamMax=[]  KbParamMin=[]  KbParamMax=[]  KtParamMin=[]  KtParamMax=[]  KbOutMin=[]  KbOutMax=[]  KtOutMin=[]  KtOutMax=[]  IntegratorOutMin=[]  IntegratorOutMax=[]  FilterOutMin=[]  FilterOutMax=[]  SumI1OutMin=[]  SumI1OutMax=[]  SumI2OutMin=[]  SumI2OutMax=[]  SumI3OutMin=[]  SumI3OutMax=[]  SumI4OutMin=[]  SumI4OutMax=[]  SumDOutMin=[]  SumDOutMax=[]  DifferentiatorOutMin=[]  DifferentiatorOutMax=[]  FilterDiffOutCoefMin=[]  FilterDiffOutCoefMax=[]  ReciprocalOutMin=[]  ReciprocalOutMax=[]  SumDenOutMin=[]  SumDenOutMax=[]  SumNumOutMin=[]  SumNumOutMax=[]  DivideOutMin=[]  DivideOutMax=[]  UdiffTsProdOutMin=[]  UdiffTsProdOutMax=[]  NTsProdOutMin=[]  NTsProdOutMax=[]  UintegralTsProdOutMin=[]  UintegralTsProdOutMax=[]  UngainTsProdOutMin=[]  UngainTsProdOutMax=[]  IntegratorContinuousStateAttributes=''  IntegratorStateMustResolveToSignalObject=off  IntegratorRTWStateStorageClass=Auto  FilterContinuousStateAttributes=''  FilterStateMustResolveToSignalObject=off  FilterRTWStateStorageClass=Auto  ParallelPVariant=InternalParameters  IdealPVariant=Disabled  IVariant=Disabled  DVariant=InternalParameters  IntegratorVariant=Disabled  SatVariant=Disabled  AWVariant=Disabled  PCopyVariant=Disabled  TRVariant=Disabled  FdbkBlocksVariant=Forward  IdealPFdbkVariant=Disabled  SatFdbkVariant=Disabled  DerivativeFilterVariant=ForwardEulerFilter  NVariant=InternalParameters  NCopyVariant=Disabled  FilterICVariant=InternalICsFilter  IntegratorICVariant=Disabled  ExternalResetVariant=Disabled  TRSumVariant=Passthrough  SumFdbkVariant=Disabled  SumVariant=Sum_PD  TsampFilterVariant=InternalTs  TsampNgainVariant=Passthrough  TsampIntegralVariant=Disabled_SignalSpec  ExternalSaturationOutDataTypeStr=Inherit: Same as second input
  Product : Product
  Subtract3 : Sum
  Sum : Sum  Inputs=|+-
  Sum3 : Sum  Inputs=|-+
  Switch1 : Switch  Threshold=25
  To Host File : quarc_library/Sinks/To Host/To Host File  file_name=CAR_12_Desired.mat  variable_name=CAR_12_Desired  decimation=1  sample_time=-1  file_format=MAT-file v.4  options=No header or footer  append=off  final_file_name=CAR_12_Desired.mat  bitrate=2000000
  To Host File1 : quarc_library/Sinks/To Host/To Host File  file_name=CAR_12_obtained.mat  variable_name=CAR_12_obtained  decimation=1  sample_time=-1  file_format=MAT-file v.4  options=No header or footer  append=off  final_file_name=CAR_12_obtained.mat  bitrate=2000000
  To calculate Intial Condition : Subsystem
  Out1 : Outport
  th2_out : Outport  Port=2
  wires:
  To calculate Intial Condition/1(Out1) -> Subtract3/2
  Sum3/1 -> PID Controller3/1
  Product/1 -> Subtract3/1
  Constant2/1 -> Sum/2
  Switch1/1 -> Product/2
  Subtract3/1 -> To Host File/1, Sum3/1
  Sum/1 -> Switch1/1
  Dividing by Radius/1 -> Product/1
  wd/1 -> Dividing by Radius/1
  Clock1/1 -> Sum/1, Switch1/3, Switch1/2
  PID Controller3/1 -> Out1/1
  th2/1 -> To Host File1/1, Sum3/2, th2_out/1

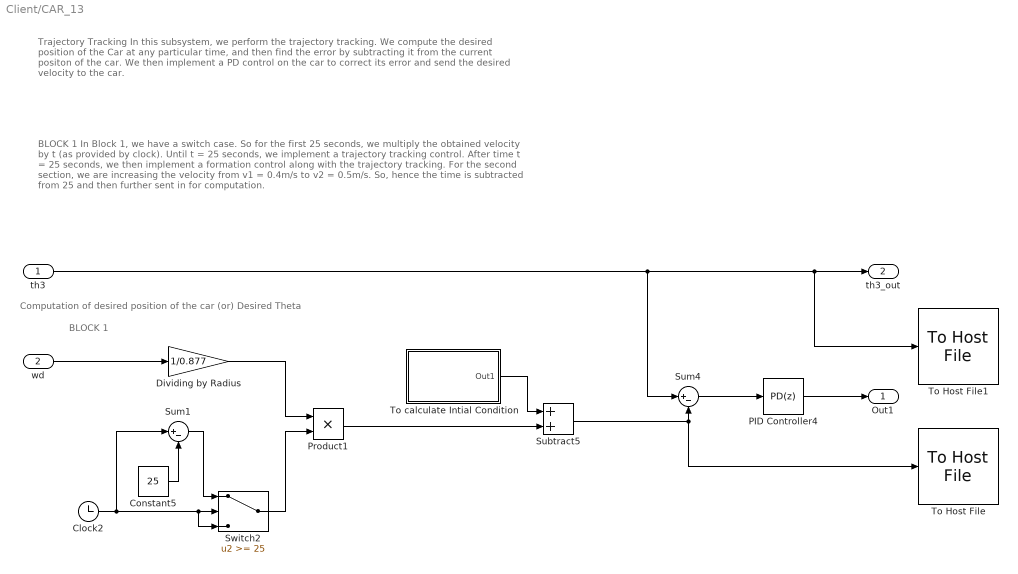
== system Client/CAR_13 ==
  note: Trajectory Tracking
      | In this subsystem, we perform the trajectory tracking.
      | We compute the desired position of the Car at any particular time, and then find the error by subtracting it from the current positon of the car.
      | We then implement a PD control on the car to correct its error and send the desired velocity to the car.
  note: BLOCK 1
  note: BLOCK 1
      | In Block 1, we have a switch case.
      | So for the first 25 seconds, we multiply the obtained velocity by t (as provided by clock). Until t = 25 seconds, we implement a trajectory tracking control.
      | After time t = 25 seconds, we then implement a formation control along with the trajectory tracking.
      | For the second section, we are increasing the velocity from v1 = 0.4m/s to v2 = 0.5m/s.
      | So, hence the time is subtracted from 25 and then further sent in for computation.
  note: Computation of desired position of the car (or) Desired Theta
  th3 : Inport
  wd : Inport  Port=2
  Clock2 : Clock
  Constant5 : Constant  Value=25
  Dividing by Radius : Gain  Gain=1/0.877
  PID Controller4 : pid_lib/PID Controller  Controller=PD  Form=Parallel  TimeDomain=Discrete-time  UseExternalTs=off  SampleTime=-1  IntegratorMethod=Forward Euler  FilterMethod=Forward Euler  ControllerParametersSource=internal  P=-0.68  I=-0.5  D=-1.75  UseFilter=on  N=1  TunerSelectOption=Transfer Function Based (PID Tuner App)  InitialConditionSource=internal  InitialConditionForIntegrator=0  InitialConditionForFilter=0  DifferentiatorICPrevScaledInput=0  ExternalReset=none  TrackingMode=off  Kt=1  LimitOutput=off  SatLimitsSource=internal  UpperSaturationLimit=inf  LowerSaturationLimit=-inf  LinearizeAsGain=on  AntiWindupMode=none  Kb=1  POutMin=[]  POutMax=[]  IOutMin=[]  IOutMax=[]  DOutMin=[]  DOutMax=[]  NOutMin=[]  NOutMax=[]  SumOutMin=[]  SumOutMax=[]  SaturationOutMin=[]  SaturationOutMax=[]  PParamMin=[]  PParamMax=[]  IParamMin=[]  IParamMax=[]  DParamMin=[]  DParamMax=[]  NParamMin=[]  NParamMax=[]  KbParamMin=[]  KbParamMax=[]  KtParamMin=[]  KtParamMax=[]  KbOutMin=[]  KbOutMax=[]  KtOutMin=[]  KtOutMax=[]  IntegratorOutMin=[]  IntegratorOutMax=[]  FilterOutMin=[]  FilterOutMax=[]  SumI1OutMin=[]  SumI1OutMax=[]  SumI2OutMin=[]  SumI2OutMax=[]  SumI3OutMin=[]  SumI3OutMax=[]  SumI4OutMin=[]  SumI4OutMax=[]  SumDOutMin=[]  SumDOutMax=[]  DifferentiatorOutMin=[]  DifferentiatorOutMax=[]  FilterDiffOutCoefMin=[]  FilterDiffOutCoefMax=[]  ReciprocalOutMin=[]  ReciprocalOutMax=[]  SumDenOutMin=[]  SumDenOutMax=[]  SumNumOutMin=[]  SumNumOutMax=[]  DivideOutMin=[]  DivideOutMax=[]  UdiffTsProdOutMin=[]  UdiffTsProdOutMax=[]  NTsProdOutMin=[]  NTsProdOutMax=[]  UintegralTsProdOutMin=[]  UintegralTsProdOutMax=[]  UngainTsProdOutMin=[]  UngainTsProdOutMax=[]  IntegratorContinuousStateAttributes=''  IntegratorStateMustResolveToSignalObject=off  IntegratorRTWStateStorageClass=Auto  FilterContinuousStateAttributes=''  FilterStateMustResolveToSignalObject=off  FilterRTWStateStorageClass=Auto  ParallelPVariant=InternalParameters  IdealPVariant=Disabled  IVariant=Disabled  DVariant=InternalParameters  IntegratorVariant=Disabled  SatVariant=Disabled  AWVariant=Disabled  PCopyVariant=Disabled  TRVariant=Disabled  FdbkBlocksVariant=Forward  IdealPFdbkVariant=Disabled  SatFdbkVariant=Disabled  DerivativeFilterVariant=ForwardEulerFilter  NVariant=InternalParameters  NCopyVariant=Disabled  FilterICVariant=InternalICsFilter  IntegratorICVariant=Disabled  ExternalResetVariant=Disabled  TRSumVariant=Passthrough  SumFdbkVariant=Disabled  SumVariant=Sum_PD  TsampFilterVariant=InternalTs  TsampNgainVariant=Passthrough  TsampIntegralVariant=Disabled_SignalSpec  ExternalSaturationOutDataTypeStr=Inherit: Same as second input
  Product1 : Product
  Subtract5 : Sum
  Sum1 : Sum  Inputs=|+-
  Sum4 : Sum  Inputs=|+-
  Switch2 : Switch  Threshold=25
  To Host File : quarc_library/Sinks/To Host/To Host File  file_name=CAR_13_Desired.mat  variable_name=CAR_13_Desired  decimation=1  sample_time=-1  file_format=MAT-file v.4  options=No header or footer  append=off  final_file_name=CAR_13_Desired.mat  bitrate=2000000
  To Host File1 : quarc_library/Sinks/To Host/To Host File  file_name=CAR_13_obtained.mat  variable_name=CAR_13_obtained  decimation=1  sample_time=-1  file_format=MAT-file v.4  options=No header or footer  append=off  final_file_name=CAR_13_obtained.mat  bitrate=2000000
  To calculate Intial Condition : Subsystem
  Out1 : Outport
  th3_out : Outport  Port=2
  wires:
  Sum4/1 -> PID Controller4/1
  Dividing by Radius/1 -> Product1/1
  To calculate Intial Condition/1(Out1) -> Subtract5/1
  Clock2/1 -> Sum1/1, Switch2/3, Switch2/2
  Sum1/1 -> Switch2/1
  wd/1 -> Dividing by Radius/1
  Constant5/1 -> Sum1/2
  PID Controller4/1 -> Out1/1
  Switch2/1 -> Product1/2
  Subtract5/1 -> To Host File/1, Sum4/2
  Product1/1 -> Subtract5/2
  th3/1 -> Sum4/1, To Host File1/1, th3_out/1

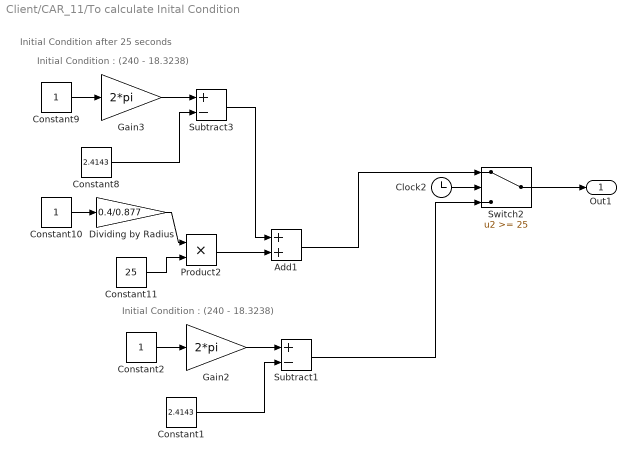
== system Client/CAR_11/To calculate Inital Condition ==
  note: Initial Condition : (240 - 18.3238)
  note: Initial Condition : (240 - 18.3238)
  note: Initial Condition after 25 seconds
  Add1 : Sum
  Clock2 : Clock
  Constant1 : Constant  Value=2.4143
  Constant10 : Constant
  Constant11 : Constant  Value=25
  Constant2 : Constant
  Constant8 : Constant  Value=2.4143
  Constant9 : Constant
  Dividing by Radius : Gain  Gain=0.4/0.877
  Gain2 : Gain  Gain=2*pi
  Gain3 : Gain  Gain=2*pi
  Product2 : Product
  Subtract1 : Sum  Inputs=+-
  Subtract3 : Sum  Inputs=+-
  Switch2 : Switch  Threshold=25
  Out1 : Outport
  wires:
  Subtract1/1 -> Switch2/3
  Switch2/1 -> Out1/1
  Clock2/1 -> Switch2/2
  Constant2/1 -> Gain2/1
  Constant1/1 -> Subtract1/2
  Gain2/1 -> Subtract1/1
  Subtract3/1 -> Add1/1
  Product2/1 -> Add1/2
  Constant8/1 -> Subtract3/2
  Constant10/1 -> Dividing by Radius/1
  Dividing by Radius/1 -> Product2/1
  Gain3/1 -> Subtract3/1
  Constant11/1 -> Product2/2
  Constant9/1 -> Gain3/1
  Add1/1 -> Switch2/1

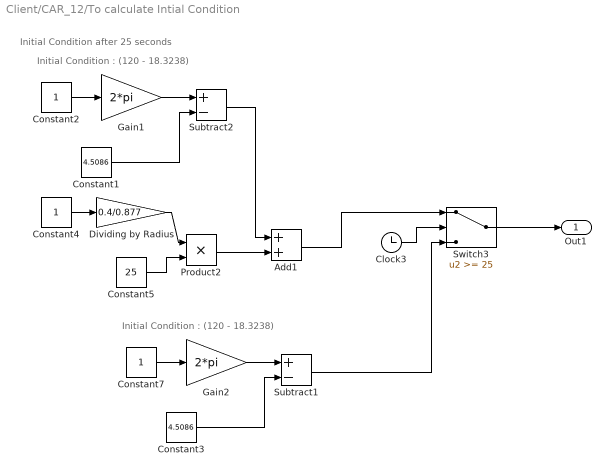
== system Client/CAR_12/To calculate Intial Condition ==
  note: Initial Condition after 25 seconds
  note: Initial Condition : (120 - 18.3238)
  note: Initial Condition : (120 - 18.3238)
  Add1 : Sum
  Clock3 : Clock
  Constant1 : Constant  Value=4.5086
  Constant2 : Constant
  Constant3 : Constant  Value=4.5086
  Constant4 : Constant
  Constant5 : Constant  Value=25
  Constant7 : Constant
  Dividing by Radius : Gain  Gain=0.4/0.877
  Gain1 : Gain  Gain=2*pi
  Gain2 : Gain  Gain=2*pi
  Product2 : Product
  Subtract1 : Sum  Inputs=+-
  Subtract2 : Sum  Inputs=+-
  Switch3 : Switch  Threshold=25
  Out1 : Outport
  wires:
  Subtract1/1 -> Switch3/3
  Clock3/1 -> Switch3/2
  Gain2/1 -> Subtract1/1
  Switch3/1 -> Out1/1
  Add1/1 -> Switch3/1
  Constant5/1 -> Product2/2
  Constant3/1 -> Subtract1/2
  Product2/1 -> Add1/2
  Dividing by Radius/1 -> Product2/1
  Constant7/1 -> Gain2/1
  Constant2/1 -> Gain1/1
  Constant1/1 -> Subtract2/2
  Gain1/1 -> Subtract2/1
  Subtract2/1 -> Add1/1
  Constant4/1 -> Dividing by Radius/1

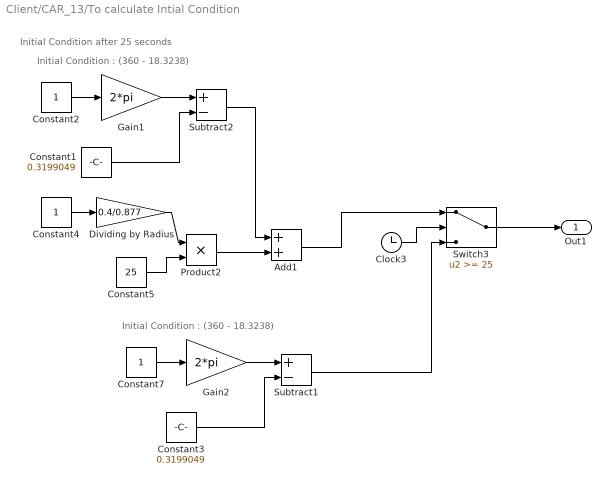
== system Client/CAR_13/To calculate Intial Condition ==
  note: Initial Condition after 25 seconds
  note: Initial Condition : (360 - 18.3238)
  note: Initial Condition : (360 - 18.3238)
  Add1 : Sum
  Clock3 : Clock
  Constant1 : Constant  Value=0.3199049
  Constant2 : Constant
  Constant3 : Constant  Value=0.3199049
  Constant4 : Constant
  Constant5 : Constant  Value=25
  Constant7 : Constant
  Dividing by Radius : Gain  Gain=0.4/0.877
  Gain1 : Gain  Gain=2*pi
  Gain2 : Gain  Gain=2*pi
  Product2 : Product
  Subtract1 : Sum  Inputs=+-
  Subtract2 : Sum  Inputs=+-
  Switch3 : Switch  Threshold=25
  Out1 : Outport
  wires:
  Subtract1/1 -> Switch3/3
  Clock3/1 -> Switch3/2
  Gain2/1 -> Subtract1/1
  Switch3/1 -> Out1/1
  Add1/1 -> Switch3/1
  Constant5/1 -> Product2/2
  Constant3/1 -> Subtract1/2
  Product2/1 -> Add1/2
  Dividing by Radius/1 -> Product2/1
  Constant7/1 -> Gain2/1
  Constant2/1 -> Gain1/1
  Constant1/1 -> Subtract2/2
  Gain1/1 -> Subtract2/1
  Subtract2/1 -> Add1/1
  Constant4/1 -> Dividing by Radius/1

== matlab function Client/CAR 12/MATLAB Function ==
  data: u input; y output; count2 data_store_memory
function y = fcn(u)
global count2
if (u>170)
    count2 = count2 + 1;
end

y = count2;

== matlab function Client/CAR 11/MATLAB Function ==
  data: u input; y output; count1 data_store_memory
function y = fcn(u)
global count1
if (u>170)
    count1 = count1 + 1;
end

y = count1;

== matlab function Client/CAR 13/MATLAB Function ==
  data: u input; y output; count3 data_store_memory
function y = fcn(u)
global count3
if (u>170)
    count3 = count3 + 1;
end

y = count3;
